simulink model "GLUINSMODEL"  (R2025a)
settings: Solver=VariableStepAuto  StartTime=0.0  StopTime=10  FixedStep=0.01  RelTol=1e-3  EnableMultiTasking=on
settings Model: Creator=cpluls  LastModifiedBy=JTerr
settings SolverCC: AlgebraicLoopSolver=TrustRegion
settings DataIOCC: LimitDataPoints=on  SaveFormat=Array  ReturnWorkspaceOutputs=off
settings OptimizationCC: LifeSpan=inf
settings DebuggingCC: UnderspecifiedInitializationDetection=Classic  MergeDetectMultiDrivingBlocksExec=none  UnconnectedInputMsg=warning  UnconnectedOutputMsg=warning  UnconnectedLineMsg=warning  StateNameClashWarn=warning  SFUnexpectedBacktrackingDiag=warning  SFNoUnconditionalDefaultTransitionDiag=warning  SFExecutionAtInitializationDiag=none  ArithmeticOperatorsInVariantConditions=warning
settings HardwareCC: ProdBitPerPointer=32.0  ProdBitPerSizeT=32.0  ProdBitPerPtrDiffT=32.0  ProdLargestAtomicFloat=None  ProdIntDivRoundTo=Undefined  ProdEndianess=Unspecified  ProdWordSize=32.0  ProdHWDeviceType=32-bit Generic
settings ModelReferenceCC: EnableRefExpFcnMdlSchedulingChecks=on  PropagateSignalLabelsOutOfModel=off
settings SFSimCC: SimUseLocalCustomCode=off  CustomCodeUndefinedFunction=UseInterfaceOnly
settings RTWCC: RTWUseLocalCustomCode=off  GPUComputeCapability=3.5  DLArmComputeVersion=19.05
settings CodeAppCC: StateflowObjectComments=on
settings GRTTargetCC: TargetLangStandard=C89/C90 (ANSI)
settings ConfigComp: CovMetricSettings=dw  CovSaveCumulativeToWorkspaceVar=on  CovSaveSingleToWorkspaceVar=on  CovExternalEMLEnable=off

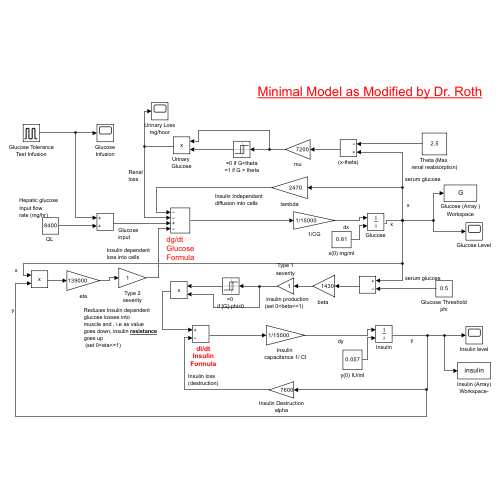
[thumbnail: Simulink's stored preview of the top-level diagram]
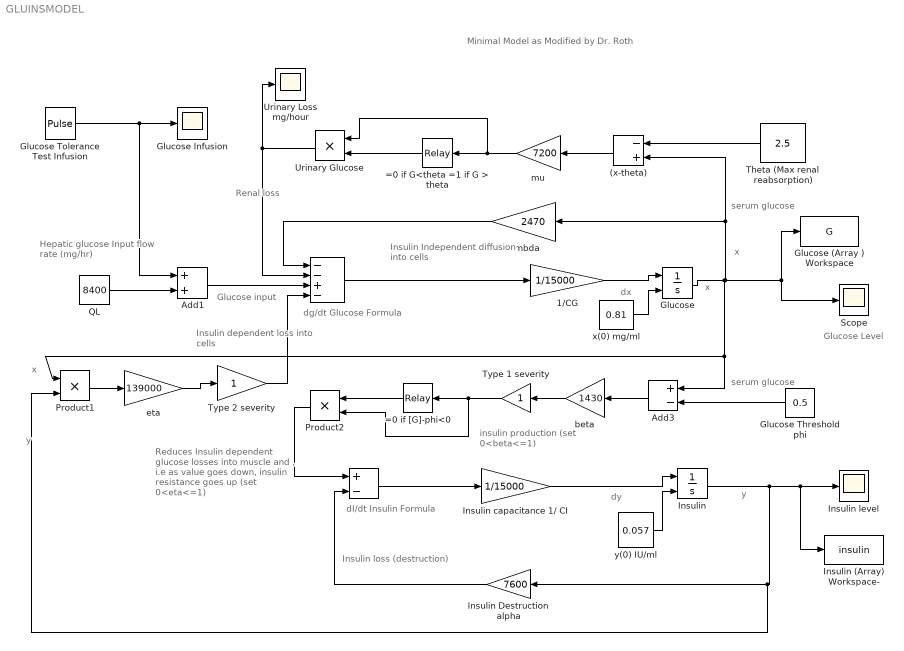
== system GLUINSMODEL ==
  note: Glucose Level
  note: dg/dt
      | Glucose
      | Formula
  note: Minimal Model as Modified by Dr. Roth
  note: dI/dt
      | Insulin
      | Formula
  note: Hepatic glucose
      | Input flow
      | rate (mg/hr)
  note: insulin production
      | (set 0<beta<=1)
  note: Reduces Insulin dependent
      | glucose losses into
      | muscle and , i.e as value
      | goes down, insulin resistance
      | goes up
      | (set 0<eta<=1)
  note: Insulin loss
      | (destruction)
  note: serum glucose
  note: Glucose
      | input
  note: Insulin dependent
      | loss into cells
  note: y
  note: x
  note: Insulin Independent
      | diffusion into cells
  note: x
  note: Renal
      | loss
  note: dy
  note: y
  note: dx
  note: x
  note: serum glucose
  " " : Sum  Inputs=--+-
  " " : Sum  Inputs=+-
  (x-theta) : Sum  Inputs=-+
  1/CG : Gain  Gain=1/15000
  =0 if [G]-phi<0 : Relay  OnSwitchValue=0  OffSwitchValue=-0.0001
  =0 if G<theta =1 if G > theta : Relay  OnSwitchValue=0  OffSwitchValue=-0.00001
  Add1 : Sum
  Add3 : Sum  Inputs=+-
  Glucose : Integrator  InitialConditionSource=external  InitialCondition=0.81
  Glucose Infusion : Scope
      settings: ActiveDisplayYMinimum=-1  ActiveDisplayYMaximum=1  DataLoggingVariableName=Ut  DataLoggingSaveFormat=Array
  Glucose (Array ) Workspace : ToWorkspace  VariableName=G  SampleTime=-1
  Glucose Threshold phi : Constant  Value=0.5
  Glucose Tolerance Test Infusion : DiscretePulseGenerator  PulseType=Time based  Amplitude=0  Period=10  PulseWidth=5
  Insulin : Integrator  InitialConditionSource=external  InitialCondition=0.057
  Insulin capacitance 1/ CI : Gain  Gain=1/15000
  Insulin (Array) Workspace- : ToWorkspace  VariableName=insulin  SampleTime=-1
  Insulin Destruction alpha : Gain  Gain=7600
  Insulin level : Scope
      settings: ActiveDisplayYMinimum=0.05694  ActiveDisplayYMaximum=0.05757  DataLoggingVariableName=I  DataLoggingSaveFormat=Array
  Product1 : Product
  Product2 : Product
  "QL " : Constant  Value=8400
  Scope : Scope
      settings: ActiveDisplayYMinimum=0.80338  ActiveDisplayYMaximum=0.81074
  Theta (Max renal reabsorption) : Constant  Value=2.5
  Type 1 severity : Gain
  Type 2 severity : Gain
  Urinary Glucose : Product
  Urinary Loss mg/hour : Scope
      settings: ActiveDisplayYMinimum=-1  ActiveDisplayYMaximum=1
  "beta " : Gain  Gain=1430
  "eta " : Gain  Gain=139000
  lambda : Gain  Gain=2470
  mu : Gain  Gain=7200
  x(0) mg/ml : Constant  Value=0.81
  y(0) IU/ml : Constant  Value=0.057
  wires:
  1/CG/1 -> Glucose/1
  Theta (Max renal reabsorption)/1 -> (x-theta)/1
  mu/1 -> Urinary Glucose/1, =0 if G<theta =1 if G > theta/1
  (x-theta)/1 -> mu/1
  Glucose/1 -> Product1/1, Add3/1, Scope/1, Glucose (Array ) Workspace/1, (x-theta)/2, lambda/1
  =0 if G<theta =1 if G > theta/1 -> Urinary Glucose/2
  Urinary Glucose/1 -> " "/2, Urinary Loss mg/hour/1
  lambda/1 -> " "/1
  " "/1 -> 1/CG/1
  "QL "/1 -> Add1/2
  Add1/1 -> " "/3
  Product1/1 -> "eta "/1
  Insulin capacitance 1/ CI/1 -> Insulin/1
  Insulin/1 -> Product1/2, Insulin Destruction alpha/1, Insulin (Array) Workspace-/1, Insulin level/1
  " "/1 -> Insulin capacitance 1/ CI/1
  Insulin Destruction alpha/1 -> " "/2
  Glucose Threshold phi/1 -> Add3/2
  =0 if [G]-phi<0/1 -> Product2/1
  Product2/1 -> " "/1
  "eta "/1 -> Type 2 severity/1
  Type 2 severity/1 -> " "/4
  Add3/1 -> "beta "/1
  "beta "/1 -> Type 1 severity/1
  Type 1 severity/1 -> Product2/2, =0 if [G]-phi<0/1
  y(0) IU/ml/1 -> Insulin/2
  x(0) mg/ml/1 -> Glucose/2
  Glucose Tolerance Test Infusion/1 -> Add1/1, Glucose Infusion/1
